simulink model "SF105A_MotCurrRegVltgLimr"  (R2013b)
settings: Solver=FixedStepDiscrete  SolverMode=SingleTasking  StartTime=0.0  StopTime=1  FixedStep=0.00025  RelTol=1e-3
undefined symbols (not defined in the file): ARCHGLBPRM_2OVERSQRT3_ULS_F32, ARCHGLBPRM_2PI_ULS_F32, BRDGVLTGHILIM_VOLT_F32, ELECGLBPRM_PWMPERDNOMX2_SEC_F32, F32TOU16OVR2PI_ULS_F32, MotCurrRegCfgCurrLoopSecOrderTrfFctEna, MotCurrRegCfgMotRVirtDax, MotCurrRegCfgMotRVirtQax, MotCurrRegVltgLimrCurrLoaScarSlewRate, MotCurrRegVltgLimrDaxAntiWdupCoeff, MotCurrRegVltgLimrDualEcuLoaScarSlewRate, MotCurrRegVltgLimrIvtrLoaScarSlewRate, MotCurrRegVltgLimrMotCurrPredEna, MotCurrRegVltgLimrMotCurrPredTi, MotCurrRegVltgLimrMotCurrQaxRefMdfnRplEna, MotCurrRegVltgLimrMotVltgBrdgFilEna, MotCurrRegVltgLimrMotVltgDaxIntglHiLim, MotCurrRegVltgLimrMotVltgDaxIntglLoLim, MotCurrRegVltgLimrMotVltgQaxFfFilEna, MotCurrRegVltgLimrMotVltgQaxIntglHiLim, MotCurrRegVltgLimrMotVltgQaxIntglLoLim, MotCurrRegVltgLimrQaxAntiWdupCoeff, MotCurrRegVltgLimrQaxAntiWdupScagDi, MotRefMdlFbCtrlDi, MotRefMdlIvtrDeadTiBrdgVltgSca, SysSt1, ZERO_VOLT_F32
libraries: NxtrLim x15, Fil x4, simulink x3, NxtrMax x2, NxtrMin x2
(part 2 of 5)

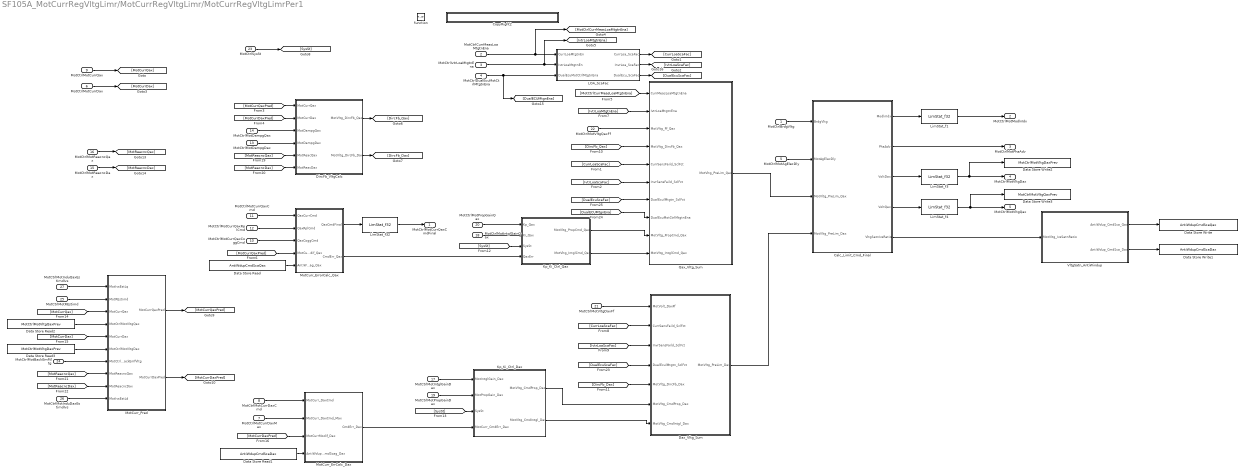
== system SF105A_MotCurrRegVltgLimr/MotCurrRegVltgLimr/MotCurrRegVltgLimrPer1 ==
  MotCtrlBrdgVltg : Inport
  MotCtrlCurrMeasLoaMtgtnEna : Inport  Port=2
  MotCtrlIvtrLoaMtgtnEna : Inport  Port=3
  MotCtrlDualEcuMotCtrlMtgtnEna : Inport  Port=4
  MotCtrlMotAgElecDly : Inport  Port=5
  MotCtrlMotCurrDax : Inport  Port=6
  MotCtrlMotCurrDaxMax : Inport  Port=7
  MotCtrlMotCurrDaxCmd : Inport  Port=8
  MotCtrlMotCurrQax : Inport  Port=9
  MotCtrlMotCurrQaxCoggCmd : Inport  Port=10
  MotCtrlMotCurrQaxCmd : Inport  Port=11
  MotCtrlMotCurrQaxRplCmd : Inport  Port=12
  MotCtrlMotDampgDax : Inport  Port=13
  MotCtrlMotDampgQax : Inport  Port=14
  MotCtrlMotReacncDax : Inport  Port=15
  MotCtrlMotReacncQax : Inport  Port=16
  MotCtrlMotIntglGainDax : Inport  Port=17
  MotCtrlMotIntglGainQax : Inport  Port=18
  MotCtrlMotPropGainDax : Inport  Port=19
  MotCtrlMotPropGainQax : Inport  Port=20
  MotCtrlMotVltgDaxFf : Inport  Port=21
  MotCtrlMotVltgQaxFf : Inport  Port=22
  MotCtrlSysSt : Inport  Port=23
  MotCtrlMotBackEmfVltg : Inport  Port=24
  "MotCtrlMotREstimd " : Inport  Port=25
  MotCtrlMotInduDaxEstimdIvs : Inport  Port=26
  MotCtrlMotInduQaxEstimdIvs : Inport  Port=27
  function : TriggerPort  TriggerType=function-call
  Calc_Limit_Cmd_Final : Subsystem
  CopyRight2 : Subsystem  Description=|  mask(Copyright Information){none=on}
      | Copyright info block.                                               
      |                                                                     
      | Place copyright information at the top of every subsystem in design.
      mask prompts: none "No parameters"
      mask help: Place copyright information at the top of every subsystem in design.
      mask Display:
      | NxtrConf = 'Nexteer Confidential';
      | 
      | sys = bdroot; %handle for the current model ("system")
      | first = get_param(sys,'Created');
      | if(isempty(first))
      |     first = datestr(now,'yyyy');
      | else
      |     first = first(end-3:end);  %year is last four digits
      | end
      | 
      | last = get_param(sys,'LastModifiedDate');
      | if isempty(last)
      |     last = datestr(now,'yyyy');
      | else
      |     last = last(end-3:end);
      | end
      | 
      | if strcmp(first,last)
      |     fprintf('%s -- Copyright %s Nexteer',NxtrConf,first)
      | else
      |     fprintf('%s -- %s%s- %s Nexteer',NxtrConf,char(169),first,last)
      | end
  Data Store Read : DataStoreRead  DataStoreName=AntiWdupCmdScaQax
  Data Store Read1 : DataStoreRead  DataStoreName=AntiWdupCmdScaDax
  Data Store Read2 : DataStoreRead  DataStoreName=MotCtrlMotVltgQaxPrev
  Data Store Read3 : DataStoreRead  DataStoreName=MotCtrlMotVltgDaxPrev
  Data Store Write : DataStoreWrite  DataStoreName=AntiWdupCmdScaQax
  Data Store Write1 : DataStoreWrite  DataStoreName=AntiWdupCmdScaDax
  Data Store Write2 : DataStoreWrite  DataStoreName=MotCtrlMotVltgDaxPrev
  Data Store Write3 : DataStoreWrite  DataStoreName=MotCtrlMotVltgQaxPrev
  Dax_Vltg_Sum : Subsystem
  DircFb_VltgCalc : Subsystem
  Kp_Ki_Ctrl_Dax : Subsystem
  Kp_Ki_Ctrl_Qax : Subsystem
  LOA_ScaFac : Subsystem
  LimStat_f1 : NxtrLim/LimStat_f32  RequirementInfo={'linktype_rmi_doors' '0000bb44 (/E-STEER Core/SubSystem Specifications/Application Functions/SF99/SF105A Current Regulator and Voltage Limiter)' '#SF105A_131' 'true' 'REQ: SF105A_131' '' } %GIDa_5b64c45d_3cb8_4503_aa08_a1be8801add7  LoLim=MOTMODLNIDXLOLIM_ULS_F32  HiLim=MOTMODLNIDXHILIM_ULS_F32
      settings: AttributesFormatString=|
      | Low Limit: %<LoLim>
      | High Limit:%<HiLim>
  LimStat_f3 : NxtrLim/LimStat_f32  RequirementInfo={'linktype_rmi_doors' '0000bb44 (/E-STEER Core/SubSystem Specifications/Application Functions/SF99/SF105A Current Regulator and Voltage Limiter)' '#SF105A_131' 'true' 'REQ: SF105A_131' '' } %GIDa_8680302d_e840_4ac4_b59c_87c18badb04a  LoLim=MOTVLTGDQAXLOLIM_VOLT_F32  HiLim=MOTVLTGDQAXHILIM_VOLT_F32
      settings: AttributesFormatString=|
      | Low Limit: %<LoLim>
      | High Limit:%<HiLim>
  LimStat_f32 : NxtrLim/LimStat_f32  RequirementInfo={'linktype_rmi_doors' '0000bb44 (/E-STEER Core/SubSystem Specifications/Application Functions/SF99/SF105A Current Regulator and Voltage Limiter)' '#SF105A_131' 'true' 'REQ: SF105A_131' '' } %GIDa_6c6b8d90_e99a_4080_8c4c_409ee69ab06d  LoLim=MOTCURRLOLIM_AMPR_F32  HiLim=MOTCURRHILIM_AMPR_F32
      settings: AttributesFormatString=|
      | Low Limit: %<LoLim>
      | High Limit:%<HiLim>
  LimStat_f4 : NxtrLim/LimStat_f32  RequirementInfo={'linktype_rmi_doors' '0000bb44 (/E-STEER Core/SubSystem Specifications/Application Functions/SF99/SF105A Current Regulator and Voltage Limiter)' '#SF105A_131' 'true' 'REQ: SF105A_131' '' } %GIDa_6dbc15d0_ee83_49e2_ba5d_de01d4cc5077  LoLim=MOTVLTGDQAXLOLIM_VOLT_F32  HiLim=MOTVLTGDQAXHILIM_VOLT_F32
      settings: AttributesFormatString=|
      | Low Limit: %<LoLim>
      | High Limit:%<HiLim>
  MotCurr_ErrCalc_Dax : Subsystem
  MotCurr_ErrorCalc_Qax : Subsystem
  MotCurr_Pred : Subsystem
  Qax_Vltg_Sum : Subsystem
  VltgSatn_AntiWindup : Subsystem
  MotCtrlMotCurrQaxCmdFinal : Outport
  MotCtrlMotModlnIdx : Outport  Port=2
  MotCtrlMotPhaAdv : Outport  Port=3
  MotCtrlMotVltgDax : Outport  Port=4
  MotCtrlMotVltgQax : Outport  Port=5
  wires:
  MotCurr_ErrorCalc_Qax/1(QaxCmdFinal) -> LimStat_f32/1
  MotCtrlMotCurrQaxCoggCmd/1 -> MotCurr_ErrorCalc_Qax/3(QaxCoggCmd)
  MotCtrlMotCurrQaxRplCmd/1 -> MotCurr_ErrorCalc_Qax/2(QaxRplCmd)
  MotCtrlMotCurrQaxCmd/1 -> MotCurr_ErrorCalc_Qax/1(QaxCurrCmd)
  MotCtrlMotCurrQax/1 -> [MotCurrQax]
  [MotCurrQaxPred] -> MotCurr_ErrorCalc_Qax/4(MotCurrModif_Qax)
  MotCurr_ErrorCalc_Qax/2(CmdErr_Qax) -> Kp_Ki_Ctrl_Qax/4(QaxErr)
  MotCtrlMotPropGainQax/1 -> Kp_Ki_Ctrl_Qax/1(Kp_Qax)
  MotCtrlMotIntglGainQax/1 -> Kp_Ki_Ctrl_Qax/2(Ki_Qax)
  MotCtrlMotVltgQaxFf/1 -> Qax_Vltg_Sum/3(MotVltg_Ff_Qax)
  Kp_Ki_Ctrl_Qax/1(MotVltg_PropCmd_Qax) -> Qax_Vltg_Sum/9(MotVltg_PropCmd_Qax)
  Kp_Ki_Ctrl_Qax/2(MotVltg_IntglCmd_Qax) -> Qax_Vltg_Sum/10(MotVltg_IntglCmd_Qax)
  MotCtrlCurrMeasLoaMtgtnEna/1 -> LOA_ScaFac/1(CurrLoaMtgtnEn), [MotCtrlCurrMeasLoaMtgtnEna]
  MotCtrlIvtrLoaMtgtnEna/1 -> LOA_ScaFac/2(IvtrLoaMtgtnEn), [IvtrLoaMtgtnEna]
  LOA_ScaFac/1(CurrLoa_ScaFac) -> [CurrLoaScaFac]
  LOA_ScaFac/2(InvrLoa_ScaFac) -> [IvtrLoaScaFac]
  [CurrLoaScaFac] -> Qax_Vltg_Sum/5(CurrSensFaild_SclFct)
  [IvtrLoaScaFac] -> Qax_Vltg_Sum/6(InvrSensFaild_SclFct)
  MotCtrlMotCurrDax/1 -> [MotCurrDax]
  [MotCurrDaxPred] -> DircFb_VltgCalc/2(MotCurrDax)
  MotCtrlMotDampgQax/1 -> DircFb_VltgCalc/3(MotDampgQax)
  MotCtrlMotDampgDax/1 -> DircFb_VltgCalc/4(MotDampgDax)
  Qax_Vltg_Sum/1(MotVltg_PreLim_Qax) -> Calc_Limit_Cmd_Final/3(MotVltg_PreLim_Qax)
  VltgSatn_AntiWindup/1(AntiWdup_CmdSca_Qax) -> Data Store Write/1
  VltgSatn_AntiWindup/2(AntiWdup_CmdSca_Dax) -> Data Store Write1/1
  [MotCurrDaxPred] -> MotCurr_ErrCalc_Dax/3(MotCurrModif_Dax)
  MotCtrlMotCurrDaxCmd/1 -> MotCurr_ErrCalc_Dax/1(MotCurr_DaxCmd)
  MotCtrlMotCurrDaxMax/1 -> MotCurr_ErrCalc_Dax/2(MotCurr_DaxCmd_Max)
  Data Store Read1/1 -> MotCurr_ErrCalc_Dax/4(AntiWdup_CmdScag_Dax)
  MotCtrlMotIntglGainDax/1 -> Kp_Ki_Ctrl_Dax/1(MotIntglGain_Dax)
  MotCtrlMotPropGainDax/1 -> Kp_Ki_Ctrl_Dax/2(MotPropGain_Dax)
  MotCurr_ErrCalc_Dax/1(CmdErr_Dax) -> Kp_Ki_Ctrl_Dax/4(MotCurr_CmdErr_Dax)
  Kp_Ki_Ctrl_Dax/2(MotVltg_CmdIntgl_Dax) -> Dax_Vltg_Sum/7(MotVltg_CmdIntgl_Dax)
  Kp_Ki_Ctrl_Dax/1(MotVltg_CmdProp_Dax) -> Dax_Vltg_Sum/6(MotVltg_CmdProp_Dax)
  MotCtrlMotVltgDaxFf/1 -> Dax_Vltg_Sum/1(MotVolt_DaxFf)
  [CurrLoaScaFac] -> Dax_Vltg_Sum/2(CurrSensFaild_SclFct)
  [IvtrLoaScaFac] -> Dax_Vltg_Sum/3(InvrSensFaild_SclFct)
  MotCtrlBrdgVltg/1 -> Calc_Limit_Cmd_Final/1(BrdgVltg)
  MotCtrlMotAgElecDly/1 -> Calc_Limit_Cmd_Final/2(MotAgElecDly)
  Dax_Vltg_Sum/1(MotVltg_PreLim_Dax) -> Calc_Limit_Cmd_Final/4(MotVltg_PreLim_Dax)
  Calc_Limit_Cmd_Final/1(ModlnIdx) -> LimStat_f1/1
  Calc_Limit_Cmd_Final/3(VoltDax) -> LimStat_f3/1
  Calc_Limit_Cmd_Final/4(VoltQax) -> LimStat_f4/1
  Calc_Limit_Cmd_Final/5(VltgSatnIvsRatio) -> VltgSatn_AntiWindup/1(MotVltg_IvsSatnRatio)
  DircFb_VltgCalc/1(MotVltg_DircFb_Qax) -> [DircFb_Qax]
  DircFb_VltgCalc/2(MotVltg_DircFb_Dax) -> [DircFb_Dax]
  [DircFb_Qax] -> Qax_Vltg_Sum/4(MotVltg_DircFb_Qax)
  [DircFb_Dax] -> Dax_Vltg_Sum/5(MotVltg_DircFb_Dax)
  MotCtrlSysSt/1 -> [SysSt]
  [SysSt] -> Kp_Ki_Ctrl_Qax/3(SysSt)
  [SysSt] -> Kp_Ki_Ctrl_Dax/3(SysSt)
  Data Store Read/1 -> MotCurr_ErrorCalc_Qax/5(AntiWdup_CmdScag_Qax)
  LimStat_f32/1 -> MotCtrlMotCurrQaxCmdFinal/1
  LimStat_f1/1 -> MotCtrlMotModlnIdx/1
  Calc_Limit_Cmd_Final/2(PhaAdv) -> MotCtrlMotPhaAdv/1
  LimStat_f3/1 -> Data Store Write2/1, MotCtrlMotVltgDax/1
  LimStat_f4/1 -> Data Store Write3/1, MotCtrlMotVltgQax/1
  [IvtrLoaMtgtnEna] -> Qax_Vltg_Sum/2(IvtrLoaMtgtnEna)
  [MotCtrlCurrMeasLoaMtgtnEna] -> Qax_Vltg_Sum/1(CurrMeasLoaMtgtnEna)
  MotCurr_Pred/1(MotCurrQaxPred) -> [MotCurrQaxPred]
  MotCurr_Pred/2(MotCurrDaxPred) -> [MotCurrDaxPred]
  [MotCurrQax] -> MotCurr_Pred/3(MotCurrQax)
  [MotCurrDax] -> MotCurr_Pred/5(MotCurrDax)
  Data Store Read3/1 -> MotCurr_Pred/6(MotCtrlMotVltgDax)
  Data Store Read2/1 -> MotCurr_Pred/4(MotCtrlMotVltgQax)
  MotCtrlMotBackEmfVltg/1 -> MotCurr_Pred/7(MotCtrlMotBackEmfVltg)
  [MotCurrQaxPred] -> DircFb_VltgCalc/1(MotCurrQax)
  "MotCtrlMotREstimd "/1 -> MotCurr_Pred/2(MotREstimd)
  MotCtrlMotInduQaxEstimdIvs/1 -> MotCurr_Pred/1(MotIvsEstLq)
  MotCtrlMotReacncQax/1 -> [MotReacncQax]
  MotCtrlMotReacncDax/1 -> [MotReacncDax]
  [MotReacncQax] -> DircFb_VltgCalc/5(MotReacQax)
  [MotReacncDax] -> DircFb_VltgCalc/6(MotReacDax)
  [MotReacncQax] -> MotCurr_Pred/8(MotReacncQax)
  [MotReacncDax] -> MotCurr_Pred/9(MotReacncDax)
  MotCtrlMotInduDaxEstimdIvs/1 -> MotCurr_Pred/10(MotIvsEstLd)
  MotCtrlDualEcuMotCtrlMtgtnEna/1 -> LOA_ScaFac/3(DualEcuMotCtrlMtgtnEna), [DualECUMtgnEna]
  [DualEcuScaFac] -> Dax_Vltg_Sum/4(DualEculMtgtn_SclFct)
  [DualECUMtgnEna] -> Qax_Vltg_Sum/8(DualEcuMotCtrlMtgtnEna)
  LOA_ScaFac/3(DualEcu_ScaFac) -> [DualEcuScaFac]
  [DualEcuScaFac] -> Qax_Vltg_Sum/7(DualEculMtgtn_SclFct)

== system SF105A_MotCurrRegVltgLimr/MotCurrRegVltgLimr/MotCurrRegVltgLimrInit1/CopyRight2 ==

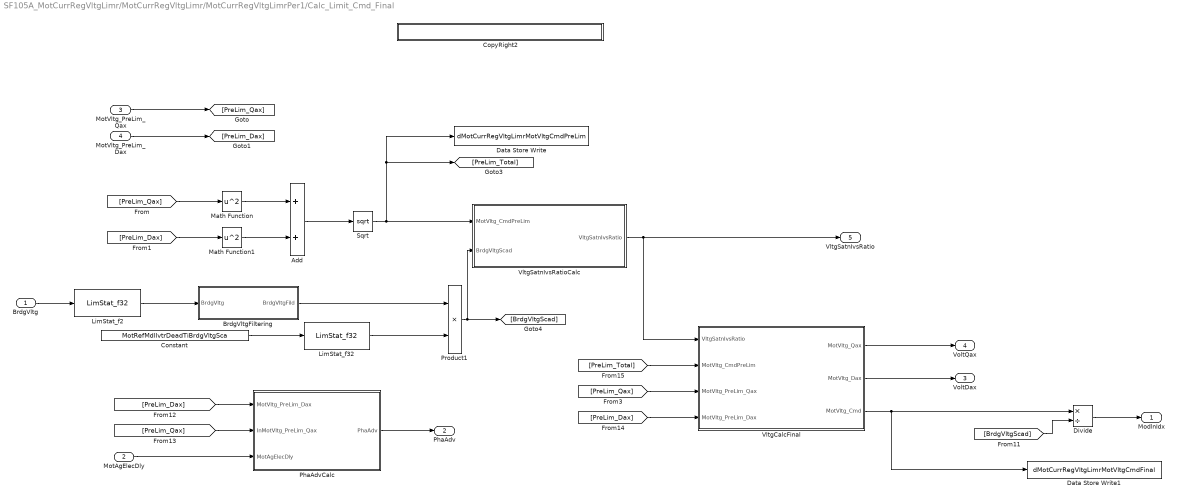
== system SF105A_MotCurrRegVltgLimr/MotCurrRegVltgLimr/MotCurrRegVltgLimrPer1/Calc_Limit_Cmd_Final ==
  BrdgVltg : Inport
  MotAgElecDly : Inport  Port=2
  MotVltg_PreLim_Qax : Inport  Port=3
  MotVltg_PreLim_Dax : Inport  Port=4
  Add : Sum  RequirementInfo={'linktype_rmi_doors' '0000bb44 (/E-STEER Core/SubSystem Specifications/Application Functions/SF99/SF105A Current Regulator and Voltage Limiter)' '#SF105A_116' 'true' 'REQ: SF105A_116' '' } %GIDa_184bcc03_5a29_4675_8bd2_076af0631f40
  BrdgVltgFiltering : Subsystem
  Constant : Constant  RequirementInfo={'linktype_rmi_doors' '0000bb44 (/E-STEER Core/SubSystem Specifications/Application Functions/SF99/SF105A Current Regulator and Voltage Limiter)' '#SF105A_115' 'true' 'REQ: SF105A_115' '' } %GIDa_1b431b0d_d8fa_4924_8a7e_96b16117a4c4  Value=MotRefMdlIvtrDeadTiBrdgVltgSca
  CopyRight2 : Subsystem  Description=|  mask(Copyright Information){none=on}
      | Copyright info block.                                               
      |                                                                     
      | Place copyright information at the top of every subsystem in design.
      mask prompts: none "No parameters"
      mask help: Place copyright information at the top of every subsystem in design.
      mask Display:
      | NxtrConf = 'Nexteer Confidential';
      | 
      | sys = bdroot; %handle for the current model ("system")
      | first = get_param(sys,'Created');
      | if(isempty(first))
      |     first = datestr(now,'yyyy');
      | else
      |     first = first(end-3:end);  %year is last four digits
      | end
      | 
      | last = get_param(sys,'LastModifiedDate');
      | if isempty(last)
      |     last = datestr(now,'yyyy');
      | else
      |     last = last(end-3:end);
      | end
      | 
      | if strcmp(first,last)
      |     fprintf('%s -- Copyright %s Nexteer',NxtrConf,first)
      | else
      |     fprintf('%s -- %s%s- %s Nexteer',NxtrConf,char(169),first,last)
      | end
  Data Store Write : DataStoreWrite  DataStoreName=dMotCurrRegVltgLimrMotVltgCmdPreLim
  Data Store Write1 : DataStoreWrite  DataStoreName=dMotCurrRegVltgLimrMotVltgCmdFinal
  Divide : Product  RequirementInfo={'linktype_rmi_doors' '0000bb44 (/E-STEER Core/SubSystem Specifications/Application Functions/SF99/SF105A Current Regulator and Voltage Limiter)' '#SF105A_120' 'true' 'REQ: SF105A_120' '' } %GIDa_633f8997_9a0c_4920_a6bc_d4d89e4d140e  Inputs=*/
  LimStat_f2 : NxtrLim/LimStat_f32  RequirementInfo={'linktype_rmi_doors' '0000bb44 (/E-STEER Core/SubSystem Specifications/Application Functions/SF99/SF105A Current Regulator and Voltage Limiter)' '#SF105A_162' 'true' 'REQ: SF105A_162' '' } %GIDa_a08859cf_e9b5_40c1_ab88_2d5ca9fa9bd6  LoLim=BRDGVLTGLOLIM_VOLT_F32  HiLim=BRDGVLTGHILIM_VOLT_F32
      settings: AttributesFormatString=|
      | LoLim: %<LoLim>
      | HiLim: %<HiLim>
  LimStat_f32 : NxtrLim/LimStat_f32  RequirementInfo={'linktype_rmi_doors' '0000bb44 (/E-STEER Core/SubSystem Specifications/Application Functions/SF99/SF105A Current Regulator and Voltage Limiter)' '#SF105A_115' 'true' 'REQ: SF105A_115' '' } %GIDa_b0dcf6af_f440_4910_84e4_7b2fd8d9492c  LoLim=MOTREFMDL_INVTERDEADTIBRDGVLTGSCALOLIM_ULS_F32  HiLim=MOTREFMDL_INVTERDEADTIBRDGVLTGSCAHILIM_ULS_F32
      settings: AttributesFormatString=|
      | LoLim: %<LoLim>
      | HiLim:%<HiLim>
  Math Function : Math  RequirementInfo={'linktype_rmi_doors' '0000bb44 (/E-STEER Core/SubSystem Specifications/Application Functions/SF99/SF105A Current Regulator and Voltage Limiter)' '#SF105A_116' 'true' 'REQ: SF105A_116' '' } %GIDa_2e28be3b_0e30_45a5_8f0c_851039ac0589  Operator=square  SaturateOnIntegerOverflow=on
  Math Function1 : Math  RequirementInfo={'linktype_rmi_doors' '0000bb44 (/E-STEER Core/SubSystem Specifications/Application Functions/SF99/SF105A Current Regulator and Voltage Limiter)' '#SF105A_116' 'true' 'REQ: SF105A_116' '' } %GIDa_1ee2d847_4428_4034_83e7_fc14e994769b  Operator=square  SaturateOnIntegerOverflow=on
  PhaAdvCalc : Subsystem
  Product1 : Product  RequirementInfo={'linktype_rmi_doors' '0000bb44 (/E-STEER Core/SubSystem Specifications/Application Functions/SF99/SF105A Current Regulator and Voltage Limiter)' '#SF105A_115' 'true' 'REQ: SF105A_115' '' } %GIDa_99f22107_0631_404a_806c_98a05cfd4301  RndMeth=Zero
  Sqrt : Sqrt  RequirementInfo={'linktype_rmi_doors' '0000bb44 (/E-STEER Core/SubSystem Specifications/Application Functions/SF99/SF105A Current Regulator and Voltage Limiter)' '#SF105A_116' 'true' 'REQ: SF105A_116' '' } %GIDa_d5330afa_b4cc_4f4a_8b77_406ea4a99f97  SaturateOnIntegerOverflow=on
  VltgCalcFinal : Subsystem  RequirementInfo={'linktype_rmi_doors' '0000bb44 (/E-STEER Core/SubSystem Specifications/Application Functions/SF99/SF105A Current Regulator and Voltage Limiter)' '#SF105A_120' 'true' 'REQ: SF105A_120' '' } %GIDa_494c122d_5837_4965_9db5_09e356f695d9
  VltgSatnIvsRatioCalc : Subsystem  RequirementInfo={'linktype_rmi_doors' '0000bb44 (/E-STEER Core/SubSystem Specifications/Application Functions/SF99/SF105A Current Regulator and Voltage Limiter)' '#SF105A_171' 'true' 'REQ: SF105A_171' '' } %GIDa_e4381c48_95db_489e_80a7_3dccc815e559
  ModlnIdx : Outport
  PhaAdv : Outport  Port=2
  VoltDax : Outport  Port=3
  VoltQax : Outport  Port=4
  VltgSatnIvsRatio : Outport  Port=5
  wires:
  Constant/1 -> LimStat_f32/1
  [PreLim_Qax] -> Math Function/1
  [PreLim_Dax] -> Math Function1/1
  Math Function/1 -> Add/1
  Math Function1/1 -> Add/2
  Add/1 -> Sqrt/1
  Sqrt/1 -> VltgSatnIvsRatioCalc/1(MotVltg_CmdPreLim), Data Store Write/1, [PreLim_Total]
  MotVltg_PreLim_Qax/1 -> [PreLim_Qax]
  MotVltg_PreLim_Dax/1 -> [PreLim_Dax]
  BrdgVltg/1 -> LimStat_f2/1
  Product1/1 -> [BrdgVltgScad], VltgSatnIvsRatioCalc/2(BrdgVltgScad)
  VltgCalcFinal/3(MotVltg_Cmd) -> Divide/1, Data Store Write1/1
  [BrdgVltgScad] -> Divide/2
  Divide/1 -> ModlnIdx/1
  LimStat_f2/1 -> BrdgVltgFiltering/1(BrdgVltg)
  LimStat_f32/1 -> Product1/2
  VltgSatnIvsRatioCalc/1(VltgSatnIvsRatio) -> VltgCalcFinal/1(VltgSatnIvsRatio), VltgSatnIvsRatio/1
  [PreLim_Qax] -> VltgCalcFinal/3(MotVltg_PreLim_Qax)
  [PreLim_Dax] -> VltgCalcFinal/4(MotVltg_PreLim_Dax)
  [PreLim_Total] -> VltgCalcFinal/2(MotVltg_CmdPreLim)
  VltgCalcFinal/1(MotVltg_Qax) -> VoltQax/1
  VltgCalcFinal/2(MotVltg_Dax) -> VoltDax/1
  [PreLim_Dax] -> PhaAdvCalc/1(MotVltg_PreLim_Dax)
  [PreLim_Qax] -> PhaAdvCalc/2(InMotVltg_PreLim_Qax)
  MotAgElecDly/1 -> PhaAdvCalc/3(MotAgElecDly)
  PhaAdvCalc/1(PhaAdv) -> PhaAdv/1
  BrdgVltgFiltering/1(BrdgVltgFild) -> Product1/1

== system SF105A_MotCurrRegVltgLimr/MotCurrRegVltgLimr/MotCurrRegVltgLimrPer1/CopyRight2 ==

== system SF105A_MotCurrRegVltgLimr/MotCurrRegVltgLimr/MotCurrRegVltgLimrPer1/Dax_Vltg_Sum ==
  MotVolt_DaxFf : Inport  RequirementInfo={'linktype_rmi_doors' '0000bb44 (/E-STEER Core/SubSystem Specifications/Application Functions/SF99/SF105A Current Regulator and Voltage Limiter)' '#SF105A_111' 'true' 'REQ: SF105A_111' '' } %GIDa_608efc51_7f85_4e44_9446_fc2a169b86cd
  CurrSensFaild_SclFct : Inport  RequirementInfo={'linktype_rmi_doors' '0000bb44 (/E-STEER Core/SubSystem Specifications/Application Functions/SF99/SF105A Current Regulator and Voltage Limiter)' '#SF105A_111' 'true' 'REQ: SF105A_111' '' } %GIDa_5c72f851_df82_41e7_8781_9d0eab3ac411  Port=2
  InvrSensFaild_SclFct : Inport  RequirementInfo={'linktype_rmi_doors' '0000bb44 (/E-STEER Core/SubSystem Specifications/Application Functions/SF99/SF105A Current Regulator and Voltage Limiter)' '#SF105A_111' 'true' 'REQ: SF105A_111' '' } %GIDa_6314902c_e0b2_4a9f_8d43_96233a1b696b  Port=3
  DualEculMtgtn_SclFct : Inport  RequirementInfo={'linktype_rmi_doors' '0000bb44 (/E-STEER Core/SubSystem Specifications/Application Functions/SF99/SF105A Current Regulator and Voltage Limiter)' '#SF105A_111' 'true' 'REQ: SF105A_111' '' } %GIDa_efeee418_0fd3_4d33_a560_39a7c4fa22b4  Port=4
  MotVltg_DircFb_Dax : Inport  RequirementInfo={'linktype_rmi_doors' '0000bb44 (/E-STEER Core/SubSystem Specifications/Application Functions/SF99/SF105A Current Regulator and Voltage Limiter)' '#SF105A_111' 'true' 'REQ: SF105A_111' '' } %GIDa_0dc38894_b516_4903_a9a7_189acd8e2b47  Port=5
  MotVltg_CmdProp_Dax : Inport  RequirementInfo={'linktype_rmi_doors' '0000bb44 (/E-STEER Core/SubSystem Specifications/Application Functions/SF99/SF105A Current Regulator and Voltage Limiter)' '#SF105A_111' 'true' 'REQ: SF105A_111' '' } %GIDa_4f2078f5_a573_476b_8ab6_5702a27071c0  Port=6
  MotVltg_CmdIntgl_Dax : Inport  RequirementInfo={'linktype_rmi_doors' '0000bb44 (/E-STEER Core/SubSystem Specifications/Application Functions/SF99/SF105A Current Regulator and Voltage Limiter)' '#SF105A_111' 'true' 'REQ: SF105A_111' '' } %GIDa_f1cdf708_b3fc_45d4_818f_e89fca6106dc  Port=7
  Add : Sum  RequirementInfo={'linktype_rmi_doors' '0000bb44 (/E-STEER Core/SubSystem Specifications/Application Functions/SF99/SF105A Current Regulator and Voltage Limiter)' '#SF105A_111' 'true' 'REQ: SF105A_111' '' } %GIDa_013e733b_bf54_44e9_8e0d_70b0bf9a3cba  Inputs=+++
  Add1 : Sum  RequirementInfo={'linktype_rmi_doors' '0000bb44 (/E-STEER Core/SubSystem Specifications/Application Functions/SF99/SF105A Current Regulator and Voltage Limiter)' '#SF105A_111' 'true' 'REQ: SF105A_111' '' } %GIDa_46f76fc9_8cd7_4a30_bd8f_695a412b3ae5
  CopyRight2 : Subsystem  Description=|  mask(Copyright Information){none=on}
      | Copyright info block.                                               
      |                                                                     
      | Place copyright information at the top of every subsystem in design.
      mask prompts: none "No parameters"
      mask help: Place copyright information at the top of every subsystem in design.
      mask Display:
      | NxtrConf = 'Nexteer Confidential';
      | 
      | sys = bdroot; %handle for the current model ("system")
      | first = get_param(sys,'Created');
      | if(isempty(first))
      |     first = datestr(now,'yyyy');
      | else
      |     first = first(end-3:end);  %year is last four digits
      | end
      | 
      | last = get_param(sys,'LastModifiedDate');
      | if isempty(last)
      |     last = datestr(now,'yyyy');
      | else
      |     last = last(end-3:end);
      | end
      | 
      | if strcmp(first,last)
      |     fprintf('%s -- Copyright %s Nexteer',NxtrConf,first)
      | else
      |     fprintf('%s -- %s%s- %s Nexteer',NxtrConf,char(169),first,last)
      | end
  Data Store Write : DataStoreWrite  DataStoreName=dMotCurrRegVltgLimrMotVltgPreLimDax
  Data Store Write1 : DataStoreWrite  DataStoreName=dMotCurrRegVltgLimrMotVltgDaxFb
  Product : Product  RequirementInfo={'linktype_rmi_doors' '0000bb44 (/E-STEER Core/SubSystem Specifications/Application Functions/SF99/SF105A Current Regulator and Voltage Limiter)' '#SF105A_111' 'true' 'REQ: SF105A_111' '' } %GIDa_14da7820_0954_431e_9cc4_f48d6ad0e238  Inputs=4
  MotVltg_PreLim_Dax : Outport  RequirementInfo={'linktype_rmi_doors' '0000bb44 (/E-STEER Core/SubSystem Specifications/Application Functions/SF99/SF105A Current Regulator and Voltage Limiter)' '#SF105A_111' 'true' 'REQ: SF105A_111' '' } %GIDa_e5ff59fa_e7e0_4785_8266_c0aa81946beb
  wires:
  MotVltg_DircFb_Dax/1 -> Add/3
  Add/1 -> Product/1
  CurrSensFaild_SclFct/1 -> Product/2
  InvrSensFaild_SclFct/1 -> Product/3
  MotVltg_CmdIntgl_Dax/1 -> Add/1
  MotVltg_CmdProp_Dax/1 -> Add/2
  Add1/1 -> Data Store Write/1, MotVltg_PreLim_Dax/1
  MotVolt_DaxFf/1 -> Add1/2
  Product/1 -> Data Store Write1/1, Add1/1
  DualEculMtgtn_SclFct/1 -> Product/4

== system SF105A_MotCurrRegVltgLimr/MotCurrRegVltgLimr/MotCurrRegVltgLimrPer1/DircFb_VltgCalc ==
  MotCurrQax : Inport
  MotCurrDax : Inport  Port=2
  MotDampgQax : Inport  Port=3
  MotDampgDax : Inport  Port=4
  MotReacQax : Inport  Port=5
  MotReacDax : Inport  Port=6
  Calculate Direct Feedback : Subsystem  TreatAsAtomicUnit=on
  Constant3 : Constant  RequirementInfo={'linktype_rmi_doors' '0000bb44 (/E-STEER Core/SubSystem Specifications/Application Functions/SF99/SF105A Current Regulator and Voltage Limiter)' '#SF105A_89' 'true' 'REQ: SF105A_89' '' ; 'linktype_rmi_doors' '0000bb44 (/E-STEER Core/SubSystem Specifications/Application Functions/SF99/SF105A Current Regulator and Voltage Limiter)' '#SF105A_94' 'true' 'REQ: SF105A_94' '' } %GIDa_1ea6686e_12cb_4464_8e76_1207af075ce1  Value=MotRefMdlFbCtrlDi
  Constant6 : Constant  RequirementInfo={'linktype_rmi_doors' '0000bb44 (/E-STEER Core/SubSystem Specifications/Application Functions/SF99/SF105A Current Regulator and Voltage Limiter)' '#SF105A_94' 'true' 'REQ: SF105A_94' '' } %GIDa_1d0a88d2_1ef9_452b_8df9_aa7b5649b20c  Value=ZERO_VOLT_F32  OutDataTypeStr=single
  CopyRight2 : Subsystem  Description=|  mask(Copyright Information){none=on}
      | Copyright info block.                                               
      |                                                                     
      | Place copyright information at the top of every subsystem in design.
      mask prompts: none "No parameters"
      mask help: Place copyright information at the top of every subsystem in design.
      mask Display:
      | NxtrConf = 'Nexteer Confidential';
      | 
      | sys = bdroot; %handle for the current model ("system")
      | first = get_param(sys,'Created');
      | if(isempty(first))
      |     first = datestr(now,'yyyy');
      | else
      |     first = first(end-3:end);  %year is last four digits
      | end
      | 
      | last = get_param(sys,'LastModifiedDate');
      | if isempty(last)
      |     last = datestr(now,'yyyy');
      | else
      |     last = last(end-3:end);
      | end
      | 
      | if strcmp(first,last)
      |     fprintf('%s -- Copyright %s Nexteer',NxtrConf,first)
      | else
      |     fprintf('%s -- %s%s- %s Nexteer',NxtrConf,char(169),first,last)
      | end
  Data Store Write : DataStoreWrite  DataStoreName=dMotCurrRegVltgLimrMotVltgDircFbQax
  Data Store Write1 : DataStoreWrite  DataStoreName=dMotCurrRegVltgLimrMotVltgDircFbDax
  If1 : If  RequirementInfo={'linktype_rmi_doors' '0000bb44 (/E-STEER Core/SubSystem Specifications/Application Functions/SF99/SF105A Current Regulator and Voltage Limiter)' '#SF105A_94' 'true' 'REQ: SF105A_94' '' } %GIDa_16eaf6ee_047b_4119_a126_ed928a6d1818  IfExpression=u1 == 1
  Merge : Merge
  Merge1 : Merge
  Zero Direct Feedback : Subsystem  RequirementInfo={'linktype_rmi_doors' '0000bb44 (/E-STEER Core/SubSystem Specifications/Application Functions/SF99/SF105A Current Regulator and Voltage Limiter)' '#SF105A_94' 'true' 'REQ: SF105A_94' '' } %GIDa_ceeeec0c_09fc_425f_8b8c_962ca11d24d6  TreatAsAtomicUnit=on
  MotVltg_DircFb_Qax : Outport
  MotVltg_DircFb_Dax : Outport  Port=2
  wires:
  Constant3/1 -> If1/1
  If1/1 -> Zero Direct Feedback/Action
  If1/2 -> Calculate Direct Feedback/Action
  Constant6/1 -> Zero Direct Feedback/1(In1)
  Merge/1 -> Data Store Write/1, MotVltg_DircFb_Qax/1
  Zero Direct Feedback/1(Qax) -> Merge/1
  Calculate Direct Feedback/1(Qax) -> Merge/2
  Merge1/1 -> Data Store Write1/1, MotVltg_DircFb_Dax/1
  Calculate Direct Feedback/2(Dax) -> Merge1/2
  Zero Direct Feedback/2(Dax) -> Merge1/1
  MotReacDax/1 -> Calculate Direct Feedback/6(MotReacDax)
  MotReacQax/1 -> Calculate Direct Feedback/5(MotReacQax)
  MotDampgDax/1 -> Calculate Direct Feedback/4(MotDampgDax)
  MotDampgQax/1 -> Calculate Direct Feedback/3(MotDampgQax)
  MotCurrQax/1 -> Calculate Direct Feedback/1(MotCurrQax)
  MotCurrDax/1 -> Calculate Direct Feedback/2(MotCurrDax)

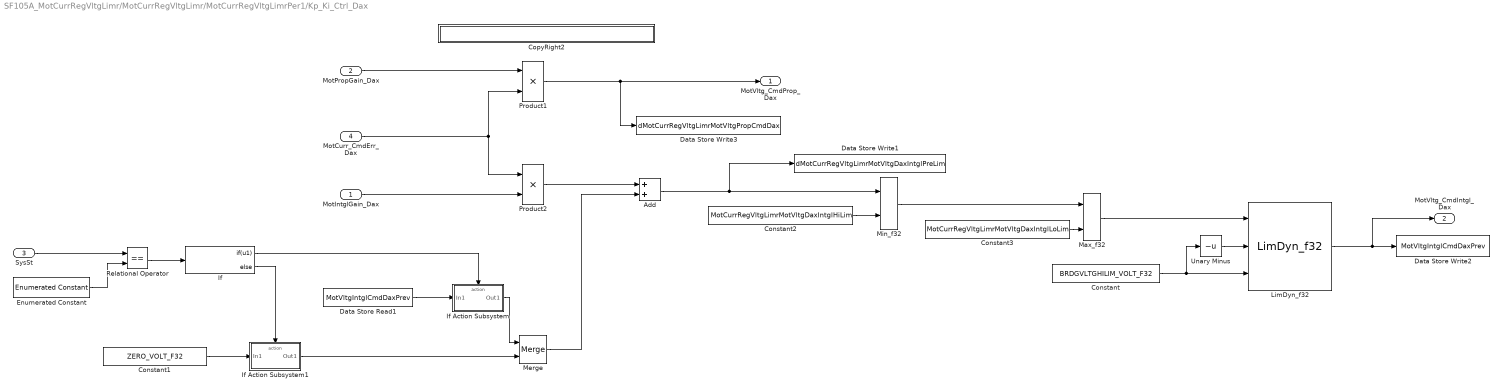
== system SF105A_MotCurrRegVltgLimr/MotCurrRegVltgLimr/MotCurrRegVltgLimrPer1/Kp_Ki_Ctrl_Dax ==
  MotIntglGain_Dax : Inport  RequirementInfo={'linktype_rmi_doors' '0000bb44 (/E-STEER Core/SubSystem Specifications/Application Functions/SF99/SF105A Current Regulator and Voltage Limiter)' '#SF105A_85' 'true' 'REQ: SF105A_85' '' } %GIDa_725c2809_bf4c_40df_8493_687ac5775410
  MotPropGain_Dax : Inport  RequirementInfo={'linktype_rmi_doors' '0000bb44 (/E-STEER Core/SubSystem Specifications/Application Functions/SF99/SF105A Current Regulator and Voltage Limiter)' '#SF105A_84' 'true' 'REQ: SF105A_84' '' } %GIDa_e4a9b43a_641d_4887_816b_a62f08c39253  Port=2
  SysSt : Inport  RequirementInfo={'linktype_rmi_doors' '0000bb44 (/E-STEER Core/SubSystem Specifications/Application Functions/SF99/SF105A Current Regulator and Voltage Limiter)' '#SF105A_137' 'true' 'REQ: SF105A_137' '' } %GIDa_7770db25_6a06_4925_94b0_43481dd7bf25  Port=3
  MotCurr_CmdErr_Dax : Inport  RequirementInfo={'linktype_rmi_doors' '0000bb44 (/E-STEER Core/SubSystem Specifications/Application Functions/SF99/SF105A Current Regulator and Voltage Limiter)' '#SF105A_84' 'true' 'REQ: SF105A_84' '' ; 'linktype_rmi_doors' '0000bb44 (/E-STEER Core/SubSystem Specifications/Application Functions/SF99/SF105A Current Regulator and Voltage Limiter)' '#SF105A_85' 'true' 'REQ: SF105A_85' '' } %GIDa_c93ecbc8_2765_4aca_ac49_759cdd1478b9  Port=4
  Add : Sum  RequirementInfo={'linktype_rmi_doors' '0000bb44 (/E-STEER Core/SubSystem Specifications/Application Functions/SF99/SF105A Current Regulator and Voltage Limiter)' '#SF105A_85' 'true' 'REQ: SF105A_85' '' } %GIDa_917a4797_aa58_444a_97c6_28edf76a1c49
  Constant : Constant  RequirementInfo={'linktype_rmi_doors' '0000bb44 (/E-STEER Core/SubSystem Specifications/Application Functions/SF99/SF105A Current Regulator and Voltage Limiter)' '#SF105A_191' 'true' 'REQ: SF105A_191' '' } %GIDa_945a6a92_b41c_4be1_9298_7ca6c5f85695  Value=BRDGVLTGHILIM_VOLT_F32
  Constant1 : Constant  RequirementInfo={'linktype_rmi_doors' '0000bb44 (/E-STEER Core/SubSystem Specifications/Application Functions/SF99/SF105A Current Regulator and Voltage Limiter)' '#SF105A_137' 'true' 'REQ: SF105A_137' '' } %GIDa_277b4085_f937_4359_ad7e_5ab9b3a921e9  Value=ZERO_VOLT_F32  OutDataTypeStr=single
  Constant2 : Constant  RequirementInfo={'linktype_rmi_doors' '0000bb44 (/E-STEER Core/SubSystem Specifications/Application Functions/SF99/SF105A Current Regulator and Voltage Limiter)' '#SF105A_181' 'true' 'REQ: SF105A_181' '' } %GIDa_4a169242_1f2e_406a_9bde_70f9a24e454a  Value=MotCurrRegVltgLimrMotVltgDaxIntglHiLim
  Constant3 : Constant  RequirementInfo={'linktype_rmi_doors' '0000bb44 (/E-STEER Core/SubSystem Specifications/Application Functions/SF99/SF105A Current Regulator and Voltage Limiter)' '#SF105A_181' 'true' 'REQ: SF105A_181' '' } %GIDa_d4dd28bf_039a_4094_9f0a_07dbaee00e3a  Value=MotCurrRegVltgLimrMotVltgDaxIntglLoLim
  CopyRight2 : Subsystem  Description=|  mask(Copyright Information){none=on}
      | Copyright info block.                                               
      |                                                                     
      | Place copyright information at the top of every subsystem in design.
      mask prompts: none "No parameters"
      mask help: Place copyright information at the top of every subsystem in design.
      mask Display:
      | NxtrConf = 'Nexteer Confidential';
      | 
      | sys = bdroot; %handle for the current model ("system")
      | first = get_param(sys,'Created');
      | if(isempty(first))
      |     first = datestr(now,'yyyy');
      | else
      |     first = first(end-3:end);  %year is last four digits
      | end
      | 
      | last = get_param(sys,'LastModifiedDate');
      | if isempty(last)
      |     last = datestr(now,'yyyy');
      | else
      |     last = last(end-3:end);
      | end
      | 
      | if strcmp(first,last)
      |     fprintf('%s -- Copyright %s Nexteer',NxtrConf,first)
      | else
      |     fprintf('%s -- %s%s- %s Nexteer',NxtrConf,char(169),first,last)
      | end
  Data Store Read1 : DataStoreRead  RequirementInfo={'linktype_rmi_doors' '0000bb44 (/E-STEER Core/SubSystem Specifications/Application Functions/SF99/SF105A Current Regulator and Voltage Limiter)' '#SF105A_85' 'true' 'REQ: SF105A_85' '' ; 'linktype_rmi_doors' '0000bb44 (/E-STEER Core/SubSystem Specifications/Application Functions/SF99/SF105A Current Regulator and Voltage Limiter)' '#SF105A_137' 'true' 'REQ: SF105A_137' '' } %GIDa_59285df0_5d01_4fdb_b8fd_c862a10d3efd  DataStoreName=MotVltgIntglCmdDaxPrev
  Data Store Write1 : DataStoreWrite  DataStoreName=dMotCurrRegVltgLimrMotVltgDaxIntglPreLim
  Data Store Write2 : DataStoreWrite  RequirementInfo={'linktype_rmi_doors' '0000bb44 (/E-STEER Core/SubSystem Specifications/Application Functions/SF99/SF105A Current Regulator and Voltage Limiter)' '#SF105A_85' 'true' 'REQ: SF105A_85' '' ; 'linktype_rmi_doors' '0000bb44 (/E-STEER Core/SubSystem Specifications/Application Functions/SF99/SF105A Current Regulator and Voltage Limiter)' '#SF105A_137' 'true' 'REQ: SF105A_137' '' } %GIDa_c2401e91_3695_49f1_8ded_ec8a4f2e228c  DataStoreName=MotVltgIntglCmdDaxPrev
  Data Store Write3 : DataStoreWrite  DataStoreName=dMotCurrRegVltgLimrMotVltgPropCmdDax
  Enumerated Constant : simulink/Sources/Enumerated Constant  RequirementInfo={'linktype_rmi_doors' '0000bb44 (/E-STEER Core/SubSystem Specifications/Application Functions/SF99/SF105A Current Regulator and Voltage Limiter)' '#SF105A_137' 'true' 'REQ: SF105A_137' '' } %GIDa_cea9164c_a3b9_4c2d_9a5e_261e7f6ce3ed  OutDataTypeStr=Enum: SysSt1  Value=SysSt1.SYSST_ENA  SampleTime=inf
  If : If  RequirementInfo={'linktype_rmi_doors' '0000bb44 (/E-STEER Core/SubSystem Specifications/Application Functions/SF99/SF105A Current Regulator and Voltage Limiter)' '#SF105A_137' 'true' 'REQ: SF105A_137' '' } %GIDa_9517d1e8_4ac0_4700_b15e_51bd0198d5e3  IfExpression=u1
  If Action Subsystem : Subsystem  RequirementInfo={'linktype_rmi_doors' '0000bb44 (/E-STEER Core/SubSystem Specifications/Application Functions/SF99/SF105A Current Regulator and Voltage Limiter)' '#SF105A_137' 'true' 'REQ: SF105A_137' '' } %GIDa_2b0cfa38_00a1_46ac_a62e_28ba926b49f1  TreatAsAtomicUnit=on
  If Action Subsystem1 : Subsystem  RequirementInfo={'linktype_rmi_doors' '0000bb44 (/E-STEER Core/SubSystem Specifications/Application Functions/SF99/SF105A Current Regulator and Voltage Limiter)' '#SF105A_137' 'true' 'REQ: SF105A_137' '' } %GIDa_6cf093d5_83a9_4b2d_a454_79c99fe448f9  TreatAsAtomicUnit=on
  LimDyn_f32 : NxtrLim/LimDyn_f32  RequirementInfo={'linktype_rmi_doors' '0000bb44 (/E-STEER Core/SubSystem Specifications/Application Functions/SF99/SF105A Current Regulator and Voltage Limiter)' '#SF105A_191' 'true' 'REQ: SF105A_191' '' } %GIDa_be62ee3a_c339_4bda_a6d7_f6960caefbdd
  Max_f32 : NxtrMax/Max_f32  RequirementInfo={'linktype_rmi_doors' '0000bb44 (/E-STEER Core/SubSystem Specifications/Application Functions/SF99/SF105A Current Regulator and Voltage Limiter)' '#SF105A_182' 'true' 'REQ: SF105A_182' '' } %GIDa_b3bc4591_d6b7_4de3_959d_417c0c5ee2c0  SFunctionSpec=single y1 = Max_f32(single u1, single u2)
      settings: AttributesFormatString=%<Name>
  Merge : Merge  RequirementInfo={'linktype_rmi_doors' '0000bb44 (/E-STEER Core/SubSystem Specifications/Application Functions/SF99/SF105A Current Regulator and Voltage Limiter)' '#SF105A_137' 'true' 'REQ: SF105A_137' '' } %GIDa_c8cbb47a_5e2e_4956_afeb_b1353b8122ec
  Min_f32 : NxtrMin/Min_f32  RequirementInfo={'linktype_rmi_doors' '0000bb44 (/E-STEER Core/SubSystem Specifications/Application Functions/SF99/SF105A Current Regulator and Voltage Limiter)' '#SF105A_182' 'true' 'REQ: SF105A_182' '' } %GIDa_f224bc25_d038_4756_bf9b_9af4544fd3dd  SFunctionSpec=single y1 = Min_f32(single u1, single u2)
      settings: AttributesFormatString=%<Name>
  Product1 : Product  RequirementInfo={'linktype_rmi_doors' '0000bb44 (/E-STEER Core/SubSystem Specifications/Application Functions/SF99/SF105A Current Regulator and Voltage Limiter)' '#SF105A_84' 'true' 'REQ: SF105A_84' '' } %GIDa_f45d90a4_3c2e_49cf_8975_6ac515276376  RndMeth=Zero
  Product2 : Product  RequirementInfo={'linktype_rmi_doors' '0000bb44 (/E-STEER Core/SubSystem Specifications/Application Functions/SF99/SF105A Current Regulator and Voltage Limiter)' '#SF105A_85' 'true' 'REQ: SF105A_85' '' } %GIDa_785a0041_89a5_4b0b_9e5e_f55b26e28f61  RndMeth=Zero
  Relational Operator : RelationalOperator  RequirementInfo={'linktype_rmi_doors' '0000bb44 (/E-STEER Core/SubSystem Specifications/Application Functions/SF99/SF105A Current Regulator and Voltage Limiter)' '#SF105A_137' 'true' 'REQ: SF105A_137' '' } %GIDa_530af221_bade_494c_8b83_78d6b2f5d7a3  Operator===  OutDataTypeStr=boolean
  Unary Minus : UnaryMinus  RequirementInfo={'linktype_rmi_doors' '0000bb44 (/E-STEER Core/SubSystem Specifications/Application Functions/SF99/SF105A Current Regulator and Voltage Limiter)' '#SF105A_191' 'true' 'REQ: SF105A_191' '' } %GIDa_7326d666_ce48_47dd_ac64_311b0d1327f4
  MotVltg_CmdProp_Dax : Outport  RequirementInfo={'linktype_rmi_doors' '0000bb44 (/E-STEER Core/SubSystem Specifications/Application Functions/SF99/SF105A Current Regulator and Voltage Limiter)' '#SF105A_84' 'true' 'REQ: SF105A_84' '' } %GIDa_1f8faef5_7c05_4600_a512_b1512b498103
  MotVltg_CmdIntgl_Dax : Outport  RequirementInfo={'linktype_rmi_doors' '0000bb44 (/E-STEER Core/SubSystem Specifications/Application Functions/SF99/SF105A Current Regulator and Voltage Limiter)' '#SF105A_85' 'true' 'REQ: SF105A_85' '' } %GIDa_1b7bf4b9_e00c_4bfa_a32e_2b554da10ba9  Port=2
  wires:
  MotCurr_CmdErr_Dax/1 -> Product2/1, Product1/2
  MotPropGain_Dax/1 -> Product1/1
  Product1/1 -> Data Store Write3/1, MotVltg_CmdProp_Dax/1
  Product2/1 -> Add/1
  LimDyn_f32/1 -> Data Store Write2/1, MotVltg_CmdIntgl_Dax/1
  SysSt/1 -> Relational Operator/1
  Enumerated Constant/1 -> Relational Operator/2
  Relational Operator/1 -> If/1
  If/1 -> If Action Subsystem/Action
  If/2 -> If Action Subsystem1/Action
  Data Store Read1/1 -> If Action Subsystem/1(In1)
  If Action Subsystem/1(Out1) -> Merge/1
  If Action Subsystem1/1(Out1) -> Merge/2
  Constant1/1 -> If Action Subsystem1/1(In1)
  Merge/1 -> Add/2
  Add/1 -> Data Store Write1/1, Min_f32/1
  Constant2/1 -> Min_f32/2
  Constant3/1 -> Max_f32/2
  Min_f32/1 -> Max_f32/1
  Max_f32/1 -> LimDyn_f32/1
  Constant/1 -> Unary Minus/1, LimDyn_f32/3
  Unary Minus/1 -> LimDyn_f32/2
  MotIntglGain_Dax/1 -> Product2/2

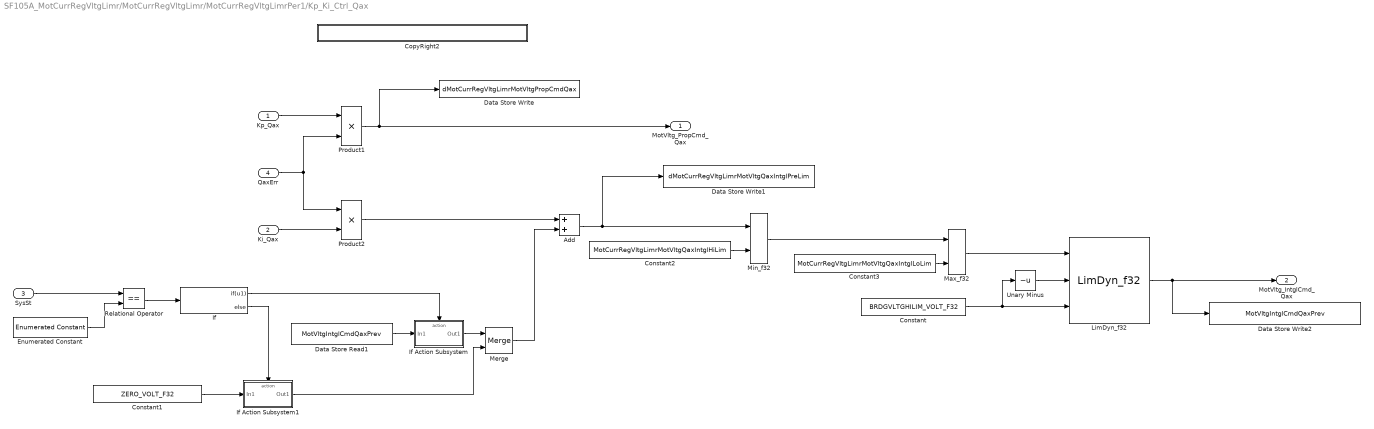
== system SF105A_MotCurrRegVltgLimr/MotCurrRegVltgLimr/MotCurrRegVltgLimrPer1/Kp_Ki_Ctrl_Qax ==
  Kp_Qax : Inport  RequirementInfo={'linktype_rmi_doors' '0000bb44 (/E-STEER Core/SubSystem Specifications/Application Functions/SF99/SF105A Current Regulator and Voltage Limiter)' '#SF105A_73' 'true' 'REQ: SF105A_73' '' } %GIDa_57e85b4c_39ca_48cc_a846_f299e689c229
  Ki_Qax : Inport  RequirementInfo={'linktype_rmi_doors' '0000bb44 (/E-STEER Core/SubSystem Specifications/Application Functions/SF99/SF105A Current Regulator and Voltage Limiter)' '#SF105A_74' 'true' 'REQ: SF105A_74' '' } %GIDa_5c26d309_3593_4eba_98d7_1516a813c20e  Port=2
  SysSt : Inport  RequirementInfo={'linktype_rmi_doors' '0000bb44 (/E-STEER Core/SubSystem Specifications/Application Functions/SF99/SF105A Current Regulator and Voltage Limiter)' '#SF105A_135' 'true' 'REQ: SF105A_135' '' } %GIDa_a406387d_a840_4bc9_90b6_78c571db18a2  Port=3
  QaxErr : Inport  RequirementInfo={'linktype_rmi_doors' '0000bb44 (/E-STEER Core/SubSystem Specifications/Application Functions/SF99/SF105A Current Regulator and Voltage Limiter)' '#SF105A_73' 'true' 'REQ: SF105A_73' '' ; 'linktype_rmi_doors' '0000bb44 (/E-STEER Core/SubSystem Specifications/Application Functions/SF99/SF105A Current Regulator and Voltage Limiter)' '#SF105A_74' 'true' 'REQ: SF105A_74' '' } %GIDa_8981aab3_9fc5_4001_81b7_c39c093ddc5f  Port=4
  Add : Sum  RequirementInfo={'linktype_rmi_doors' '0000bb44 (/E-STEER Core/SubSystem Specifications/Application Functions/SF99/SF105A Current Regulator and Voltage Limiter)' '#SF105A_74' 'true' 'REQ: SF105A_74' '' } %GIDa_4b21478b_1f9d_48a5_b52f_0b3e64d6feed
  Constant : Constant  RequirementInfo={'linktype_rmi_doors' '0000bb44 (/E-STEER Core/SubSystem Specifications/Application Functions/SF99/SF105A Current Regulator and Voltage Limiter)' '#SF105A_184' 'true' 'REQ: SF105A_184' '' } %GIDa_29629d3e_5a1a_429f_9a72_aead909d7c1c  Value=BRDGVLTGHILIM_VOLT_F32
  Constant1 : Constant  RequirementInfo={'linktype_rmi_doors' '0000bb44 (/E-STEER Core/SubSystem Specifications/Application Functions/SF99/SF105A Current Regulator and Voltage Limiter)' '#SF105A_135' 'true' 'REQ: SF105A_135' '' } %GIDa_a42ee6f0_c890_4b7f_b8af_d2e49d080707  Value=ZERO_VOLT_F32  OutDataTypeStr=single
  Constant2 : Constant  RequirementInfo={'linktype_rmi_doors' '0000bb44 (/E-STEER Core/SubSystem Specifications/Application Functions/SF99/SF105A Current Regulator and Voltage Limiter)' '#SF105A_179' 'true' 'REQ: SF105A_179' '' ; 'linktype_rmi_doors' '0000bb44 (/E-STEER Core/SubSystem Specifications/Application Functions/SF99/SF105A Current Regulator and Voltage Limiter)' '#SF105A_180' 'true' 'REQ: SF105A_180' '' } %GIDa_a79361e1_0504_40e9_8347_75407d17f493  Value=MotCurrRegVltgLimrMotVltgQaxIntglHiLim
  Constant3 : Constant  RequirementInfo={'linktype_rmi_doors' '0000bb44 (/E-STEER Core/SubSystem Specifications/Application Functions/SF99/SF105A Current Regulator and Voltage Limiter)' '#SF105A_179' 'true' 'REQ: SF105A_179' '' ; 'linktype_rmi_doors' '0000bb44 (/E-STEER Core/SubSystem Specifications/Application Functions/SF99/SF105A Current Regulator and Voltage Limiter)' '#SF105A_180' 'true' 'REQ: SF105A_180' '' } %GIDa_a5d74cd9_19bf_428c_a28f_10c4bfb0a431  Value=MotCurrRegVltgLimrMotVltgQaxIntglLoLim
  CopyRight2 : Subsystem  Description=|  mask(Copyright Information){none=on}
      | Copyright info block.                                               
      |                                                                     
      | Place copyright information at the top of every subsystem in design.
      mask prompts: none "No parameters"
      mask help: Place copyright information at the top of every subsystem in design.
      mask Display:
      | NxtrConf = 'Nexteer Confidential';
      | 
      | sys = bdroot; %handle for the current model ("system")
      | first = get_param(sys,'Created');
      | if(isempty(first))
      |     first = datestr(now,'yyyy');
      | else
      |     first = first(end-3:end);  %year is last four digits
      | end
      | 
      | last = get_param(sys,'LastModifiedDate');
      | if isempty(last)
      |     last = datestr(now,'yyyy');
      | else
      |     last = last(end-3:end);
      | end
      | 
      | if strcmp(first,last)
      |     fprintf('%s -- Copyright %s Nexteer',NxtrConf,first)
      | else
      |     fprintf('%s -- %s%s- %s Nexteer',NxtrConf,char(169),first,last)
      | end
  Data Store Read1 : DataStoreRead  RequirementInfo={'linktype_rmi_doors' '0000bb44 (/E-STEER Core/SubSystem Specifications/Application Functions/SF99/SF105A Current Regulator and Voltage Limiter)' '#SF105A_74' 'true' 'REQ: SF105A_74' '' ; 'linktype_rmi_doors' '0000bb44 (/E-STEER Core/SubSystem Specifications/Application Functions/SF99/SF105A Current Regulator and Voltage Limiter)' '#SF105A_135' 'true' 'REQ: SF105A_135' '' } %GIDa_3a3b11cb_bcd9_47e1_9499_0799ad2261ea  DataStoreName=MotVltgIntglCmdQaxPrev
  Data Store Write : DataStoreWrite  DataStoreName=dMotCurrRegVltgLimrMotVltgPropCmdQax
  Data Store Write1 : DataStoreWrite  RequirementInfo={'linktype_rmi_doors' '0000bb44 (/E-STEER Core/SubSystem Specifications/Application Functions/SF99/SF105A Current Regulator and Voltage Limiter)' '#SF105A_74' 'true' 'REQ: SF105A_74' '' ; 'linktype_rmi_doors' '0000bb44 (/E-STEER Core/SubSystem Specifications/Application Functions/SF99/SF105A Current Regulator and Voltage Limiter)' '#SF105A_135' 'true' 'REQ: SF105A_135' '' } %GIDa_73a774ff_6d03_4b0b_992d_f91e6fe2d6df  DataStoreName=dMotCurrRegVltgLimrMotVltgQaxIntglPreLim
  Data Store Write2 : DataStoreWrite  RequirementInfo={'linktype_rmi_doors' '0000bb44 (/E-STEER Core/SubSystem Specifications/Application Functions/SF99/SF105A Current Regulator and Voltage Limiter)' '#SF105A_74' 'true' 'REQ: SF105A_74' '' ; 'linktype_rmi_doors' '0000bb44 (/E-STEER Core/SubSystem Specifications/Application Functions/SF99/SF105A Current Regulator and Voltage Limiter)' '#SF105A_135' 'true' 'REQ: SF105A_135' '' } %GIDa_fec9473f_982e_4ac2_afb0_19d55f362c13  DataStoreName=MotVltgIntglCmdQaxPrev
  Enumerated Constant : simulink/Sources/Enumerated Constant  RequirementInfo={'linktype_rmi_doors' '0000bb44 (/E-STEER Core/SubSystem Specifications/Application Functions/SF99/SF105A Current Regulator and Voltage Limiter)' '#SF105A_135' 'true' 'REQ: SF105A_135' '' } %GIDa_2b310fba_2638_4ffe_93c1_23b485e16567  OutDataTypeStr=Enum: SysSt1  Value=SysSt1.SYSST_ENA  SampleTime=inf
  If : If  RequirementInfo={'linktype_rmi_doors' '0000bb44 (/E-STEER Core/SubSystem Specifications/Application Functions/SF99/SF105A Current Regulator and Voltage Limiter)' '#SF105A_135' 'true' 'REQ: SF105A_135' '' } %GIDa_ffbb68d9_7847_4d21_b8f7_d5b1410c2e58  IfExpression=u1
  If Action Subsystem : Subsystem  RequirementInfo={'linktype_rmi_doors' '0000bb44 (/E-STEER Core/SubSystem Specifications/Application Functions/SF99/SF105A Current Regulator and Voltage Limiter)' '#SF105A_135' 'true' 'REQ: SF105A_135' '' } %GIDa_af0aec57_175e_43c6_ac76_7b87820d9ffd  TreatAsAtomicUnit=on
  If Action Subsystem1 : Subsystem  RequirementInfo={'linktype_rmi_doors' '0000bb44 (/E-STEER Core/SubSystem Specifications/Application Functions/SF99/SF105A Current Regulator and Voltage Limiter)' '#SF105A_135' 'true' 'REQ: SF105A_135' '' } %GIDa_a5c89f6f_6142_4003_8af6_09a213493254  TreatAsAtomicUnit=on
  LimDyn_f32 : NxtrLim/LimDyn_f32  RequirementInfo={'linktype_rmi_doors' '0000bb44 (/E-STEER Core/SubSystem Specifications/Application Functions/SF99/SF105A Current Regulator and Voltage Limiter)' '#SF105A_184' 'true' 'REQ: SF105A_184' '' } %GIDa_b834edb9_12ea_4842_bdf5_e3a4a6d98ec2
  Max_f32 : NxtrMax/Max_f32  RequirementInfo={'linktype_rmi_doors' '0000bb44 (/E-STEER Core/SubSystem Specifications/Application Functions/SF99/SF105A Current Regulator and Voltage Limiter)' '#SF105A_179' 'true' 'REQ: SF105A_179' '' ; 'linktype_rmi_doors' '0000bb44 (/E-STEER Core/SubSystem Specifications/Application Functions/SF99/SF105A Current Regulator and Voltage Limiter)' '#SF105A_180' 'true' 'REQ: SF105A_180' '' } %GIDa_e11bb254_7c38_4bba_a7ed_4a790640eb71  SFunctionSpec=single y1 = Max_f32(single u1, single u2)
      settings: AttributesFormatString=%<Name>
  Merge : Merge  RequirementInfo={'linktype_rmi_doors' '0000bb44 (/E-STEER Core/SubSystem Specifications/Application Functions/SF99/SF105A Current Regulator and Voltage Limiter)' '#SF105A_135' 'true' 'REQ: SF105A_135' '' } %GIDa_d0e52cd1_cc9f_4de7_a730_ed7e8674e3e3
  Min_f32 : NxtrMin/Min_f32  RequirementInfo={'linktype_rmi_doors' '0000bb44 (/E-STEER Core/SubSystem Specifications/Application Functions/SF99/SF105A Current Regulator and Voltage Limiter)' '#SF105A_179' 'true' 'REQ: SF105A_179' '' ; 'linktype_rmi_doors' '0000bb44 (/E-STEER Core/SubSystem Specifications/Application Functions/SF99/SF105A Current Regulator and Voltage Limiter)' '#SF105A_180' 'true' 'REQ: SF105A_180' '' } %GIDa_b1cb7787_faf1_4bca_be72_be71b71b1b30  SFunctionSpec=single y1 = Min_f32(single u1, single u2)
      settings: AttributesFormatString=%<Name>
  Product1 : Product  RequirementInfo={'linktype_rmi_doors' '0000bb44 (/E-STEER Core/SubSystem Specifications/Application Functions/SF99/SF105A Current Regulator and Voltage Limiter)' '#SF105A_73' 'true' 'REQ: SF105A_73' '' } %GIDa_8ea8d7bb_bde8_4d56_83f9_1f2b92d26db6  RndMeth=Zero
  Product2 : Product  RequirementInfo={'linktype_rmi_doors' '0000bb44 (/E-STEER Core/SubSystem Specifications/Application Functions/SF99/SF105A Current Regulator and Voltage Limiter)' '#SF105A_74' 'true' 'REQ: SF105A_74' '' } %GIDa_72eb3fc2_57ea_497f_9a4d_ba501a7be200  RndMeth=Zero
  Relational Operator : RelationalOperator  RequirementInfo={'linktype_rmi_doors' '0000bb44 (/E-STEER Core/SubSystem Specifications/Application Functions/SF99/SF105A Current Regulator and Voltage Limiter)' '#SF105A_135' 'true' 'REQ: SF105A_135' '' } %GIDa_04d95cd2_cde3_4227_a8d0_1c35a017e746  Operator===  OutDataTypeStr=boolean
  Unary Minus : UnaryMinus  RequirementInfo={'linktype_rmi_doors' '0000bb44 (/E-STEER Core/SubSystem Specifications/Application Functions/SF99/SF105A Current Regulator and Voltage Limiter)' '#SF105A_184' 'true' 'REQ: SF105A_184' '' } %GIDa_fe1d6b82_bbc5_436f_b036_f3d0ff39e98f
  MotVltg_PropCmd_Qax : Outport  RequirementInfo={'linktype_rmi_doors' '0000bb44 (/E-STEER Core/SubSystem Specifications/Application Functions/SF99/SF105A Current Regulator and Voltage Limiter)' '#SF105A_73' 'true' 'REQ: SF105A_73' '' } %GIDa_1fa1f2f3_ce79_4075_82a4_157ca66c174f
  MotVltg_IntglCmd_Qax : Outport  RequirementInfo={'linktype_rmi_doors' '0000bb44 (/E-STEER Core/SubSystem Specifications/Application Functions/SF99/SF105A Current Regulator and Voltage Limiter)' '#SF105A_74' 'true' 'REQ: SF105A_74' '' } %GIDa_64b9357f_7272_4904_9326_c7a8ffe51b95  Port=2
  wires:
  QaxErr/1 -> Product1/2, Product2/1
  Kp_Qax/1 -> Product1/1
  Ki_Qax/1 -> Product2/2
  Product1/1 -> Data Store Write/1, MotVltg_PropCmd_Qax/1
  Product2/1 -> Add/1
  LimDyn_f32/1 -> Data Store Write2/1, MotVltg_IntglCmd_Qax/1
  SysSt/1 -> Relational Operator/1
  Enumerated Constant/1 -> Relational Operator/2
  Relational Operator/1 -> If/1
  If/1 -> If Action Subsystem/Action
  If/2 -> If Action Subsystem1/Action
  Data Store Read1/1 -> If Action Subsystem/1(In1)
  If Action Subsystem/1(Out1) -> Merge/1
  If Action Subsystem1/1(Out1) -> Merge/2
  Constant1/1 -> If Action Subsystem1/1(In1)
  Add/1 -> Data Store Write1/1, Min_f32/1
  Constant2/1 -> Min_f32/2
  Constant3/1 -> Max_f32/2
  Min_f32/1 -> Max_f32/1
  Max_f32/1 -> LimDyn_f32/1
  Merge/1 -> Add/2
  Constant/1 -> LimDyn_f32/3, Unary Minus/1
  Unary Minus/1 -> LimDyn_f32/2
